simulink model "S1_sats"  (R2025b)
settings: Solver=ode1be  StartTime=0.0  StopTime=0.5  RelTol=1e-3
values from neighbouring files (symbols this model uses):
  b1 = 1.2611    [S1_DHRL.m]    (also in S1_sat.m)
  b2 = 0.8909    [S1_DHRL.m]    (also in S1_sat.m)
  c1 = 15.0914    [S1_DHRL.m]    (also in S1_sat.m)
  c2 = 13.4548    [S1_DHRL.m]    (also in S1_sat.m)
  gamma = 0.5508    [S1_DHRL.m]    (also in S1_sat.m)
  h = 0.001    [S1_DHRL.m]    (also in S1_sat.m)
  k = 21.9999    [S1_DHRL.m]    (also in S1_sat.m)
  ks = 641.6    [S1_DHRL.m]    (also in S1_sat.m)
  Mb = 1.999*10^-4    (= 0.0001999)    [S1_DHRL.m]    (also in S1_sat.m)
undefined symbols (not defined in the file or in its folder): magnitude
libraries: fod x6
settings Model: Creator=IT7  LastModifiedBy=Wassim DJ

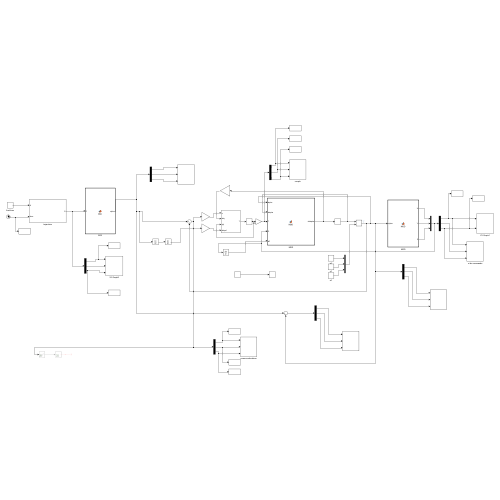
[thumbnail: Simulink's stored preview of the top-level diagram]
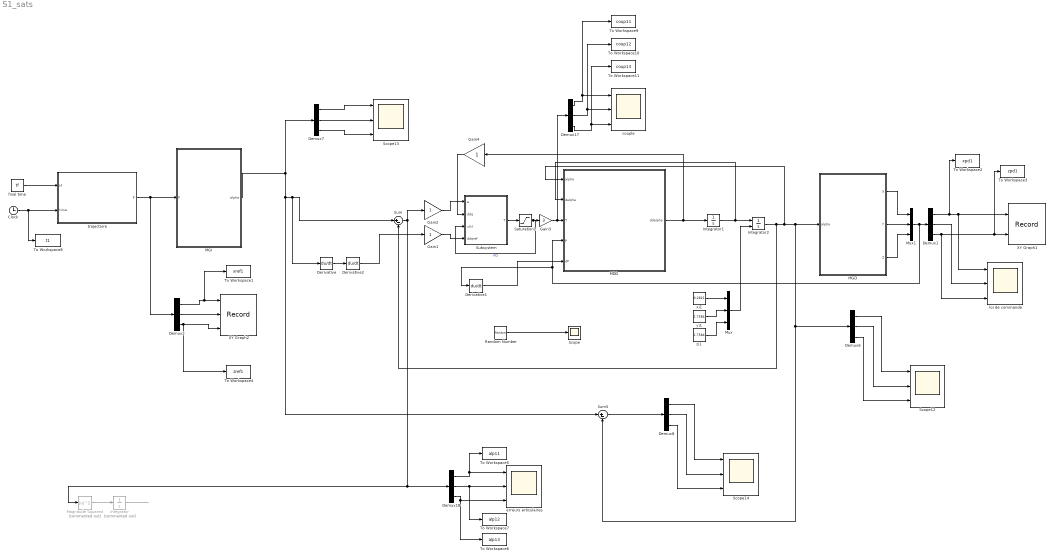
== system S1_sats ==
  Clock : Clock
  Demux{1..2,6..8,17..18} (7 alike) : Demux  Outputs=3
  Derivative : Derivative
  Derivative1 : Derivative
  Derivative2 : Derivative
  Gain1 : Gain
  Gain2 : Gain
  Gain3 : Gain  Gain=3
  Gain4 : Gain
  Integrator : Integrator  Commented=on  InitialCondition=[0 0 0]
  Integrator1 : Integrator
  Integrator2 : Integrator  InitialConditionSource=external
  MDD : MATLAB Function  TreatAsAtomicUnit=on
  MGD : MATLAB Function  TreatAsAtomicUnit=on
  MGI : MATLAB Function  TreatAsAtomicUnit=on
  Magnitude Squared : Math  Commented=on  Operator=magnitude^2
  Mux : Mux  Inputs=3
  Mux1 : Mux  Inputs=3
  Random Number : RandomNumber  Variance=0.001  Seed=4  SampleTime=0.001
  Saturation1 : Saturate  UpperLimit=15/12  LowerLimit=-15/12
  Scope : Scope
  Scope12 : Scope  NumInputPorts=3
      settings: ActiveDisplayYMinimum=-0.04767  ActiveDisplayYMaximum=2.22139  DataLoggingVariableName=ScopeData2
  Scope13 : Scope  NumInputPorts=3
      settings: ActiveDisplayYMinimum=-0.0501  ActiveDisplayYMaximum=2.21858  DataLoggingVariableName=ScopeData3
  Scope14 : Scope  NumInputPorts=3
      settings: ActiveDisplayYMinimum=-0.007  ActiveDisplayYMaximum=0.00073  DataLoggingVariableName=ScopeData4
  Subsystem : Subsystem
  Sum : Sum  Inputs=|+-
  Sum5 : Sum  Inputs=|+-
  To Workspace1 : ToWorkspace  VariableName=xref1  SampleTime=-1
      settings: Save2DSignal=2-D array (concatenate along first dimension)
  To Workspace10 : ToWorkspace  VariableName=coup12  SampleTime=-1
      settings: Save2DSignal=2-D array (concatenate along first dimension)
  To Workspace11 : ToWorkspace  VariableName=coup13  SampleTime=-1
      settings: Save2DSignal=2-D array (concatenate along first dimension)
  To Workspace2 : ToWorkspace  VariableName=xpd1  SampleTime=-1
      settings: Save2DSignal=2-D array (concatenate along first dimension)
  To Workspace3 : ToWorkspace  VariableName=zpd1  SampleTime=-1
      settings: Save2DSignal=2-D array (concatenate along first dimension)
  To Workspace4 : ToWorkspace  VariableName=zref1  SampleTime=-1
      settings: Save2DSignal=2-D array (concatenate along first dimension)
  To Workspace5 : ToWorkspace  VariableName=alp11  SampleTime=-1
      settings: Save2DSignal=2-D array (concatenate along first dimension)
  To Workspace6 : ToWorkspace  VariableName=alp13  SampleTime=-1
      settings: Save2DSignal=2-D array (concatenate along first dimension)
  To Workspace7 : ToWorkspace  VariableName=alp12  SampleTime=-1
      settings: Save2DSignal=2-D array (concatenate along first dimension)
  To Workspace8 : ToWorkspace  VariableName=t1  SampleTime=-1
      settings: Save2DSignal=2-D array (concatenate along first dimension)
  To Workspace9 : ToWorkspace  VariableName=coup11  SampleTime=-1
      settings: Save2DSignal=2-D array (concatenate along first dimension)
  XY Graph1 : Record  NumPorts=2.0  FileSettingsInternal="{\"entries\":[{\"content\":{\"excelSettings\":{\"content\":{},\"type\":\"Streamout.ExcelSettings\"},\"parquetSettings\":{\"content\":{},\"type\":\"Streamout.ParquetSettings\"}},\"type\":\"Streamout.FileSettingStorage\",\"uuid\":\"\"}],\"packageUris\":[\"http:\\/\\/schema.mathworks.com\\/mf0\\/streamout_blocks\\/R2020a\"],\"version\":\"1.0\"}"  FrameSettings=[0, 0]  Layout=[1 1]  SignalsInternal="{\"entries\":[{\"content\":{\"signals\":[{\"content\":{\"blockPath\":[],\"dimensions\":[1],\"domain\":\"\",\"lineColor\":\"#fe330a\",\"lineWidth\":2,\"port\":1,\"signalID\":1,\"signalName\":\"Demux1:1\"},\"type\":\"RecordBlkView.Signal\",\"uuid\":\"\"},{\"content\":{\"blockPath\":[],\"dimensions\":[1],\"domain\":\"\",\"lineColor\":\"#22b573\",\"lineWidth\":2,\"port\":2,\"signalID\":2,\"signalName\":\"Demux1:3\"},\"type\":\"RecordBlkView.Signal\",\"uuid\":\"\"}]},\"type\":\"RecordBlkView.InputSignals\",\"uuid\":\"\"}],\"packageUris\":[\"http:\\/\\/schema.mathworks.com\\/mf0\\/streamout_blocks\\/R2020a\"],\"version\":\"1.0\"}"  VisualizationBindings="{\"xyplotplugin\":{\"info\":[{\"series\":[],\"subplotID\":1}]}}"  CompatibilityTag=XY  st=-1
  XY Graph2 : Record  NumPorts=3.0  FileSettingsInternal="{\"entries\":[{\"content\":{\"excelSettings\":{\"content\":{},\"type\":\"Streamout.ExcelSettings\"},\"parquetSettings\":{\"content\":{},\"type\":\"Streamout.ParquetSettings\"}},\"type\":\"Streamout.FileSettingStorage\",\"uuid\":\"\"}],\"packageUris\":[\"http:\\/\\/schema.mathworks.com\\/mf0\\/streamout_blocks\\/R2020a\"],\"version\":\"1.0\"}"  FrameSettings=[0, 0, 0]  Layout=[1 1]  SignalsInternal="{\"entries\":[{\"content\":{\"signals\":[{\"content\":{\"blockPath\":[],\"dimensions\":[1,1],\"domain\":\"\",\"lineColor\":\"#0072bd\",\"lineWidth\":2,\"port\":1,\"signalID\":1,\"signalName\":\"Demux2:1\"},\"type\":\"RecordBlkView.Signal\",\"uuid\":\"\"},{\"content\":{\"blockPath\":[],\"dimensions\":[1,1],\"domain\":\"\",\"lineColor\":\"#d95319\",\"lineWidth\":2,\"port\":2,\"signalID\":2,\"signalName\":\"Demux2:2\"},\"type\":\"RecordBlkView.Signal\",\"uuid\":\"\"},{\"content\":{\"blockPath\":[],\"dimensions\":[1,1],\"domain\":\"\",\"lineColor\":\"#edb120\",\"lineWidth\":2,\"port\":3,\"signalID\":3,\"signalName\":\"Demux2:3\"},\"type\":\"RecordBlkView.Signal\",\"uuid\":\"\"}]},\"type\":\"RecordBlkView.InputSignals\",\"uuid\":\"\"}],\"packageUris\":[\"http:\\/\\/schema.mathworks.com\\/mf0\\/streamout_blocks\\/R2020a\"],\"version\":\"1.0\"}"  VisualizationBindings="{\"xyplotplugin\":{\"info\":[{\"series\":[],\"subplotID\":1}]}}"  CompatibilityTag=XY  st=-1
  couple : Scope  NumInputPorts=3
      settings: ActiveDisplayYMinimum=-10.181  ActiveDisplayYMaximum=8.9868  DataLoggingVariableName=ScopeData5
  erreurs articulaires : Scope  NumInputPorts=3
      settings: ActiveDisplayYMinimum=-0.00705  ActiveDisplayYMaximum=0.00126  DataLoggingVariableName=ScopeData6
  final time : Constant  Value=tf
  loi de commande : Scope  NumInputPorts=3
      settings: ActiveDisplayYMinimum=-0.31282  ActiveDisplayYMaximum=0.31253
  trajectoire : Subsystem
  xi1 : Constant  Value=0.2821
  yi1 : Constant  Value=1.7584
  zi1 : Constant  Value=1.7584
  wires:
  Integrator/1 -> ?
  Demux2/2 -> XY Graph2/2
  final time/1 -> trajectoire/1(tf)
  trajectoire/1(P) -> Demux2/1, MGI/1(P)
  Gain3/1 -> Demux17/1, MDD/3(T)
  Demux18/1 -> To Workspace5/1, erreurs articulaires/1
  Demux8/2 -> Scope14/2
  Demux1/1 -> XY Graph1/1, loi de commande/1, To Workspace2/1
  Magnitude Squared/1 -> Integrator/1
  Derivative1/1 -> MDD/5(dP)
  yi1/1 -> Mux/2
  Demux7/1 -> Scope13/1
  MGD/3(Z) -> Mux1/3
  Saturation1/1 -> Subsystem/3(x(t)), Gain3/1  "PD"
  Random Number/1 -> Scope/1
  Integrator2/1 -> Sum/2, MDD/1(alpha), MGD/1(alpha), Demux6/1, Sum5/2
  Demux6/3 -> Scope12/3
  Demux18/3 -> To Workspace6/1, erreurs articulaires/3
  Demux6/1 -> Scope12/1
  Demux2/1 -> To Workspace1/1, XY Graph2/1
  Derivative2/1 -> Gain1/1
  Gain4/1 -> Subsystem/2(ddq)
  Mux1/1 -> MDD/4(P), Derivative1/1, Demux1/1
  Demux2/3 -> XY Graph2/3, To Workspace4/1
  Sum5/1 -> Demux8/1
  Integrator1/1 -> MDD/2(dalpha), Integrator2/1
  Demux17/1 -> To Workspace9/1, couple/1
  Demux17/2 -> To Workspace10/1, couple/2
  MDD/1(ddalpha) -> Gain4/1, Integrator1/1
  Gain2/1 -> Subsystem/1(e)
  Demux6/2 -> Scope12/2
  Subsystem/1(T) -> Saturation1/1
  Demux17/3 -> To Workspace11/1, couple/3
  Demux1/3 -> loi de commande/3, XY Graph1/2, To Workspace3/1
  xi1/1 -> Mux/1
  Mux/1 -> Integrator2/2
  Demux8/3 -> Scope14/3
  Demux7/2 -> Scope13/2
  MGI/1(alpha) -> Derivative/1, Sum/1, Sum5/1, Demux7/1
  MGD/2(Y) -> Mux1/2
  Clock/1 -> To Workspace8/1, trajectoire/2("time ")
  MGD/1(X) -> Mux1/1
  Demux1/2 -> loi de commande/2
  Demux8/1 -> Scope14/1
  Demux18/2 -> To Workspace7/1, erreurs articulaires/2
  Demux7/3 -> Scope13/3
  Derivative/1 -> Derivative2/1
  zi1/1 -> Mux/3
  Gain1/1 -> Subsystem/4(ddqref)
  Sum/1 -> Magnitude Squared/1, Demux18/1, Gain2/1

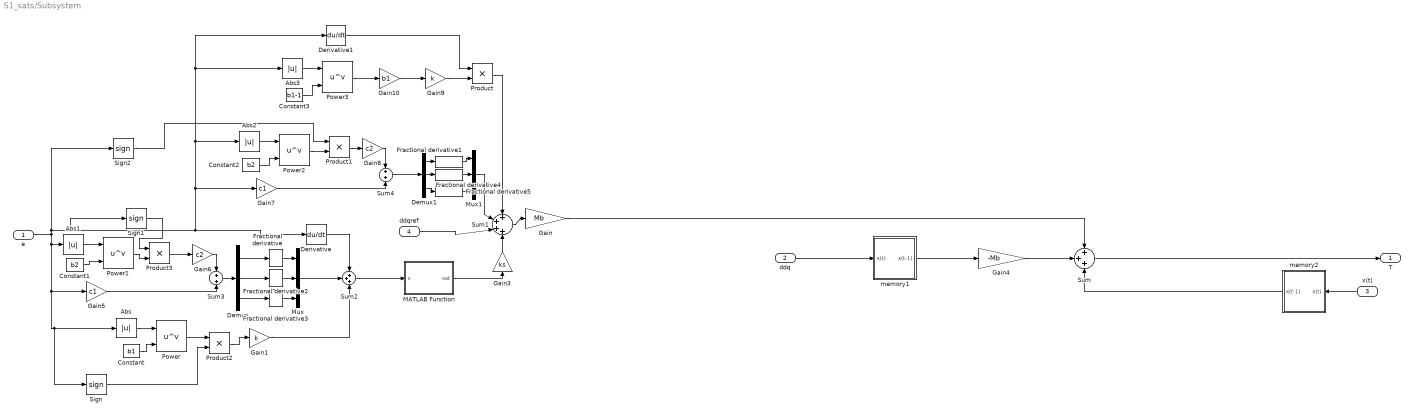
== system S1_sats/Subsystem ==
  e : Inport
  ddq : Inport  Port=2
  x(t) : Inport  Port=3
  ddqref : Inport  Port=4
  Abs{,1..3} (4 alike) : Abs  SaturateOnIntegerOverflow=off
  Constant : Constant  Value=b1
  Constant1 : Constant  Value=b2
  Constant2 : Constant  Value=b2
  Constant3 : Constant  Value=b1-1
  Demux : Demux  Outputs=3
  Demux1 : Demux  Outputs=3
  Derivative : Derivative
  Derivative1 : Derivative
  Fractional derivative : fod/Fractional derivative  gam=gamma  ww=[0.001; 1000]  n=5  nFod=off
      settings: SourceProductName=FOMCON Toolbox
  Fractional derivative1 : fod/Fractional derivative  gam=gamma+1  ww=[0.001; 1000]  n=5  nFod=off
      settings: SourceProductName=FOMCON Toolbox
  Fractional derivative2 : fod/Fractional derivative  gam=gamma  ww=[0.001; 1000]  n=5  nFod=off
      settings: SourceProductName=FOMCON Toolbox
  Fractional derivative3 : fod/Fractional derivative  gam=gamma  ww=[0.001; 1000]  n=5  nFod=off
      settings: SourceProductName=FOMCON Toolbox
  Fractional derivative4 : fod/Fractional derivative  gam=gamma+1  ww=[0.001; 1000]  n=5  nFod=off
      settings: SourceProductName=FOMCON Toolbox
  Fractional derivative5 : fod/Fractional derivative  gam=gamma+1  ww=[0.001; 1000]  n=5  nFod=off
      settings: SourceProductName=FOMCON Toolbox
  Gain : Gain  Gain=Mb
  Gain1 : Gain  Gain=k
  Gain10 : Gain  Gain=b1
  Gain3 : Gain  Gain=ks
  Gain4 : Gain  Gain=-Mb
  Gain5 : Gain  Gain=c1
  Gain6 : Gain  Gain=c2
  Gain7 : Gain  Gain=c1
  Gain8 : Gain  Gain=c2
  Gain9 : Gain  Gain=k
  MATLAB Function : MATLAB Function  TreatAsAtomicUnit=on
  Mux : Mux  Inputs=3
  Mux1 : Mux  Inputs=3
  Power{,1..3} (4 alike) : Math  Operator=pow
  Product{,1..3} (4 alike) : Product
  Sign : Signum
  Sign1 : Signum
  Sign2 : Signum
  Sum : Sum  Inputs=+++
  Sum1 : Sum  Inputs=++++
  Sum2 : Sum  Inputs=+++
  Sum3 : Sum
  Sum4 : Sum
  memory1 : Subsystem
  memory2 : Subsystem
  T : Outport
  wires:
  Derivative/1 -> Sum2/1
  ddq/1 -> memory1/1(x(t))
  Sum1/1 -> Gain/1
  Gain/1 -> Sum/1
  Gain4/1 -> Sum/2
  Abs/1 -> Power/1
  Constant/1 -> Power/2
  Power/1 -> Product2/1
  Gain1/1 -> Sum2/3
  Constant1/1 -> Power1/2
  Abs1/1 -> Power1/1
  Gain5/1 -> Sum3/2
  Gain6/1 -> Sum3/1
  Abs2/1 -> Power2/1
  Gain8/1 -> Sum4/1
  Power2/1 -> Product1/2
  Product1/1 -> Gain8/1
  Gain7/1 -> Sum4/2
  Constant2/1 -> Power2/2
  Abs3/1 -> Power3/1
  Power3/1 -> Gain10/1
  Gain10/1 -> Gain9/1
  Constant3/1 -> Power3/2
  Product/1 -> Sum1/1
  Gain9/1 -> Product/2
  Derivative1/1 -> Product/1
  Sum3/1 -> Demux/1
  Demux/1 -> Fractional derivative/1
  Demux/2 -> Fractional derivative2/1
  Demux/3 -> Fractional derivative3/1
  Fractional derivative/1 -> Mux/1
  Fractional derivative3/1 -> Mux/3
  Fractional derivative2/1 -> Mux/2
  Mux/1 -> Sum2/2
  Sum4/1 -> Demux1/1
  Demux1/1 -> Fractional derivative1/1
  Fractional derivative1/1 -> Mux1/1
  Fractional derivative4/1 -> Mux1/2
  Demux1/2 -> Fractional derivative4/1
  Fractional derivative5/1 -> Mux1/3
  Demux1/3 -> Fractional derivative5/1
  Sign2/1 -> Product1/1
  Product2/1 -> Gain1/1
  Sign/1 -> Product2/2
  Product3/1 -> Gain6/1
  Power1/1 -> Product3/2
  Sign1/1 -> Product3/1
  Mux1/1 -> Sum1/2
  e/1 -> Abs1/1, Sign/1, Abs/1, Gain5/1, Sign2/1, Sign1/1, Abs3/1, Derivative1/1, Abs2/1, Gain7/1, Derivative/1
  MATLAB Function/1(sat) -> Gain3/1
  ddqref/1 -> Sum1/3
  Gain3/1 -> Sum1/4
  Sum2/1 -> MATLAB Function/1(s)
  Sum/1 -> T/1
  x(t)/1 -> memory2/1(x(t))
  memory1/1(x(t-1)) -> Gain4/1
  memory2/1(x(t-1)) -> Sum/3

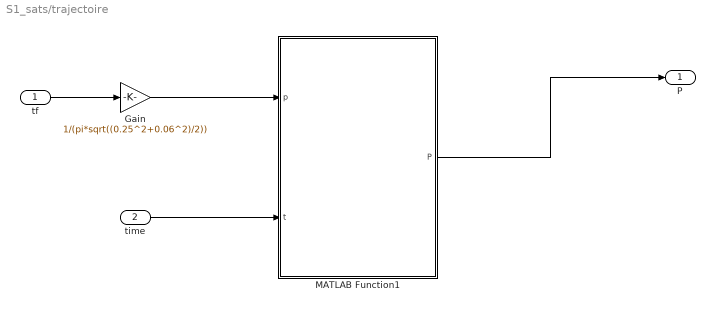
== system S1_sats/trajectoire ==
  tf : Inport
  "time " : Inport  Port=2
  Gain : Gain  Gain=1/(pi*sqrt((0.25^2+0.06^2)/2))
  MATLAB Function1 : MATLAB Function  TreatAsAtomicUnit=on
  P : Outport  VectorParamsAs1DForOutWhenUnconnected=off
  wires:
  MATLAB Function1/1(P) -> P/1
  Gain/1 -> MATLAB Function1/1(p)
  "time "/1 -> MATLAB Function1/2(t)
  tf/1 -> Gain/1

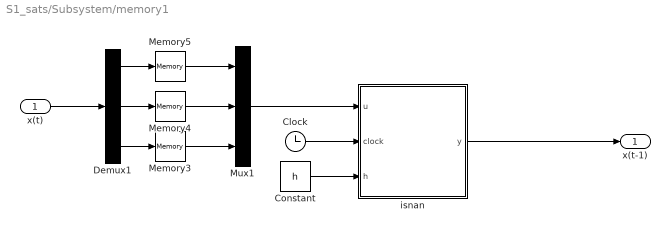
== system S1_sats/Subsystem/memory1 ==
  x(t) : Inport
  Clock : Clock
  Constant : Constant  Value=h
  Demux1 : Demux  Outputs=3
  Memory3 : Memory
  Memory4 : Memory
  Memory5 : Memory
  Mux1 : Mux  Inputs=3
  isnan : MATLAB Function  TreatAsAtomicUnit=on
  x(t-1) : Outport  VectorParamsAs1DForOutWhenUnconnected=off
  wires:
  x(t)/1 -> Demux1/1
  Demux1/1 -> Memory5/1
  Demux1/3 -> Memory3/1
  Demux1/2 -> Memory4/1
  Memory5/1 -> Mux1/1
  Memory4/1 -> Mux1/2
  Memory3/1 -> Mux1/3
  Mux1/1 -> isnan/1(u)
  isnan/1(y) -> x(t-1)/1
  Clock/1 -> isnan/2(clock)
  Constant/1 -> isnan/3(h)

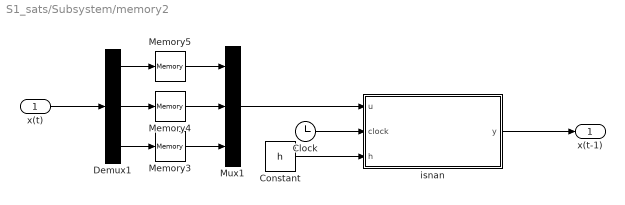
== system S1_sats/Subsystem/memory2 ==
  x(t) : Inport
  Clock : Clock
  Constant : Constant  Value=h
  Demux1 : Demux  Outputs=3
  Memory3 : Memory  InheritSampleTime=on
  Memory4 : Memory  InheritSampleTime=on
  Memory5 : Memory  InheritSampleTime=on
  Mux1 : Mux  Inputs=3
  isnan : MATLAB Function  TreatAsAtomicUnit=on
  x(t-1) : Outport  VectorParamsAs1DForOutWhenUnconnected=off
  wires:
  x(t)/1 -> Demux1/1
  Demux1/1 -> Memory5/1
  Demux1/3 -> Memory3/1
  Demux1/2 -> Memory4/1
  Memory5/1 -> Mux1/1
  Memory4/1 -> Mux1/2
  Memory3/1 -> Mux1/3
  Mux1/1 -> isnan/1(u)
  isnan/1(y) -> x(t-1)/1
  Clock/1 -> isnan/2(clock)
  Constant/1 -> isnan/3(h)

== matlab function S1_sats/MDD ==
  data: alpha input; ddalpha output; dalpha input; T input; P input; dP input
function ddalpha = MDD(alpha,dalpha,T,P,dP)
ddalpha = zeros(1,3);
phi = [0 2*pi/3 4*pi/3];
l1 = 0.205;
r = 0.15-0.024;
% these boudjedir table 2.1 page 30
mn = 0.042;
mfb = 0.028;
mb = 0.098;
mc = 0.015;
g = 9.81;
Im = 3.72e-5;
% mch=0.7;
% documentation 0
% rotation matrix
R1 = [cos(phi(1)) -sin(phi(1)) 0;sin(phi(1)) cos(phi(1)) 0;0 0 1];
R2 = [cos(phi(2)) -sin(phi(2)) 0;sin(phi(2)) cos(phi(2)) 0;0 0 1]; 
R3 = [cos(phi(3)) -sin(phi(3)) 0;sin(phi(3)) cos(phi(3)) 0;0 0 1]; 

% eq 4.4
s1 = [P(1);P(2);P(3)]-R1*([r;0;0]+[l1*cos(alpha(1));0;l1*sin(alpha(1))]);    
s2 = [P(1);P(2);P(3)]-R2*([r;0;0]+[l1*cos(alpha(2));0;l1*sin(alpha(2))]); 
s3 = [P(1);P(2);P(3)]-R3*([r;0;0]+[l1*cos(alpha(3));0;l1*sin(alpha(3))]); 

% eq 4.9
b1 = R1*[-l1*sin(alpha(1));0;l1*cos(alpha(1))];
b2 = R2*[-l1*sin(alpha(2));0;l1*cos(alpha(2))];
b3 = R3*[-l1*sin(alpha(3));0;l1*cos(alpha(3))];

% eq 4.8
ds1 = [dP(1);dP(2);dP(3)]-R1*[-l1*sin(alpha(1));0;l1*cos(alpha(1))]*dalpha(1);
ds2 = [dP(1);dP(2);dP(3)]-R2*[-l1*sin(alpha(2));0;l1*cos(alpha(2))]*dalpha(2);
ds3 = [dP(1);dP(2);dP(3)]-R3*[-l1*sin(alpha(3));0;l1*cos(alpha(3))]*dalpha(3);

db1 = R1*[-l1*cos(alpha(1));0;-l1*sin(alpha(1))]*dalpha(1);
db2 = R2*[-l1*cos(alpha(2));0;-l1*sin(alpha(2))]*dalpha(2);
db3 = R3*[-l1*cos(alpha(3));0;-l1*sin(alpha(3))]*dalpha(3);

% eq 4.13
J = inv([s1';s2';s3'])*[s1'*b1 0 0;0 s2'*b2 0;0 0 s3'*b3];

dJ = inv([s1';s2';s3'])*(-[ds1';ds2';ds3']*J+[ds1'*b1+s1'*db1 0 0;0 ds2'*b2+s2'*db2 0;0 0 ds3'*b3+s3'*db3]);
% these boudjedir
% equa 2.42
 mnt = mn+mfb ; %+mch

% equa 2.49
Tgn = J'*mnt*[0 0 -g]';

% equa 2.44
mbr = mb+mc+2/3*mfb;

% equa 2.43
rgb = l1*(1/2*mb+mc+2/3*mfb)/mbr;

% equa 2.50
Tgb = rgb*mbr*g*[cos(alpha(1)) cos(alpha(2)) cos(alpha(3))]';

% equa 2.46
Ibc = l1^2*(mb/3+mc+2/3*mfb);
% equa 2.45
Ib = (Im*12^2+Ibc)*eye(3);

% equa 2.54
 ddalpha = (inv(Ib + mnt*J'*J)*(T - J'*mnt*dJ*dalpha' + Tgn + Tgb))';
if isnan(ddalpha)
    ddalpha = zeros(1,3);
end

== matlab function S1_sats/trajectoire/MATLAB Function1 ==
  data: P output; p input; t input
function P   = trajectoire(p,t)


A=0.25;
B=0.06;
D=pi*sqrt((A^2+B^2)/2);



Xdes=0.25-A*(1-cos(pi*(t)/(p*D)));
Ydes=0*t;
Zdes=-0.43+B*sin(pi*(t)/(p*D));

dXdes=-A*pi/(p*D)*(sin(pi*(t)/(p*D)));
dYdes=0*t;
dZdes=B*pi/(p*D)*cos(pi*(t)/(p*D));

ddXdes=A*pi/(p*D)*pi/(p*D)*cos(pi*(t)/(p*D));
ddYdes=0*t;
ddZdes=-B*pi/(p*D)*pi/(p*D)*sin(pi*(t)/(p*D));

% Xdes=-0.25+A*(1-cos(pi*t/(p*D)));
% Ydes=0*t;
% Zdes=-0.43+B*sin(pi*t/(p*D));

P = [Xdes,Ydes,Zdes];
%dP = [dXdes,dYdes,dZdes];
%ddP = [ddXdes,ddYdes,ddZdes];

end

== matlab function S1_sats/Subsystem/MATLAB Function ==
  data: s input; sat output
function sat = satuaration(s)
epsilon = 10;

if abs(s) < epsilon
    sat = s/epsilon;
else
    sat = sign(s);
end

== matlab function S1_sats/MGI ==
  data: P input; alpha output
function alpha = MGI(P)
phi = [0 2*pi/3 4*pi/3];
l1 = 0.205;
l2 = 0.380;
r = 0.15-0.024;
X = P(1,1);
Y = P(1,2);
Z = P(1,3);

A = zeros(1,3);
B = 2*Z*l1;
C = zeros(1,3);

for i=1:3
A(i) = 2*r*l1-2*X*l1*cos(phi(i))-2*Y*l1*sin(phi(i));
C(i) = l2^2-l1^2-r^2-X^2-Y^2-Z^2+2*X*r*cos(phi(i))+2*Y*r*sin(phi(i));    
end

alpha = zeros(1,3);
for i=1:3
    alpha(i) =  2*atan( (2*B+sqrt(abs(4*B^2+4*(A(i)+C(i))*(A(i)-C(i)))))/(2*(A(i)+C(i))));
    alpha(i) = double(alpha(i));
end

== matlab function S1_sats/MGD ==
  data: alpha input; X output; Y output; Z output
function [X,Y,Z]  = MGD(alpha)

phi = [0 2*pi/3 4*pi/3];
l1 = 0.205;
l2 = 0.380;
r = 0.15-0.024;

D = zeros(1,3);
E = zeros(1,3);
F = zeros(1,3);
G = zeros(1,3);

for i=1:3
   D(i)=-l2^2+l1^2+r^2+2*r*l1*cos(alpha(i));
   E(i)=2*(r+l1*cos(alpha(i)))*cos(phi(i));
   F(i)=2*(r+l1*cos(alpha(i)))*sin(phi(i));
   G(i)=-2*l1*sin(alpha(i))  ;
end
% H1 = -(E(3)-E(1))*(G(2)-G(1))+(G(3)-G(1))*(E(2)-E(1));
% H2 = -(F(3)-F(1))*(E(2)-E(1))+(E(3)-E(1))*(F(2)-F(1));
% H3 = -(D(3)-D(1))*(E(2)-E(1))+(E(3)-E(1))*(D(2)-D(1));
% H4 = (D(3)-D(1))*(F(2)-F(1))-(F(3)-F(1))*(D(1)-D(2));
% H5 = -(G(3)-G(1))*(F(2)-F(1))-(F(3)-F(1))*(G(1)-G(2));

H1 = E(1)*G(2)-E(1)*G(3)-E(2)*G(1)+E(2)*G(3)+E(3)*G(1)-E(3)*G(2);
H2 = E(1)*(-F(2)+F(3))+E(2)*(F(1)-F(3))+E(3)*(-F(1)+F(2));
H3 = E(1)*(-D(2)+D(3))+E(2)*(D(1)-D(3))+E(3)*(-D(1)+D(2));
H4 = F(1)*(D(2)-D(3))+F(2)*(-D(1)+D(3))+F(3)*(D(1)-D(2));
H5 = F(1)*(-G(2)+G(3))+F(2)*(G(1)-G(3))+F(3)*(-G(1)+G(2));

L = ((H5^2+H1^2)/(H2^2))+1;
M = 2*(H5*H4+H1*H3)/(H2^2)-(H5*E(1)+H1*F(1))/H2-G(1);
N = (H4^2+H3^2)/H2^2-(H4*E(1)+H3*F(1))/H2+D(1);
Z = min((-M+sqrt(abs(M^2-4*L*N)))/(2*L),(-M-sqrt(abs(M^2-4*L*N)))/(2*L));
X = Z*(H5/H2)+(H4/H2);
Y = Z*(H1/H2)+(H3/H2);

X = double(X);
Y = double(Y);
Z = double(Z);

== matlab function S1_sats/Subsystem/memory2/isnan ==
  data: u input; y output; clock input; h input
function y = fcn(u,clock,h)
y = zeros(length(u),1);
for i = 1:3
if isnan(u(i)) || clock/h < 3
    y(i) = 0; 
else 
   y(i) = u(i);
end
end

== matlab function S1_sats/Subsystem/memory1/isnan ==
  data: u input; y output; clock input; h input
function y = fcn(u,clock,h)
y = zeros(length(u),1);
for i = 1:3
if isnan(u(i)) || clock/h < 3
    y(i) = 0; 
else 
   y(i) = u(i);
end
end
